simulink library "csc_tup_time_update_lib"  (R2014b)
settings: Solver=ode45  SolverMode=SingleTasking  StartTime=0.0  StopTime=10.0  RelTol=1e-3
undefined symbols (not defined in the file or in its folder): fcv_initializing
libraries: simulink x1, util_info_lib x1, csc_fcv_filter_convergence_lib x1, csu_itu_inertial_time_update_lib x1, csu_ttu_topo_time_update_lib x1, util_common_lib x1
settings Model: ExtModeAutoUpdateStatusClock=off  Creator=escrane  LastModifiedBy=mstewart

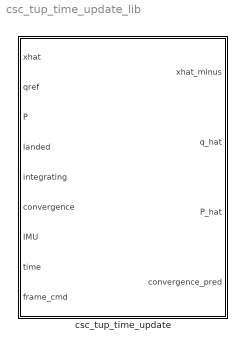
== system csc_tup_time_update_lib ==
  csc_tup_time_update : Subsystem

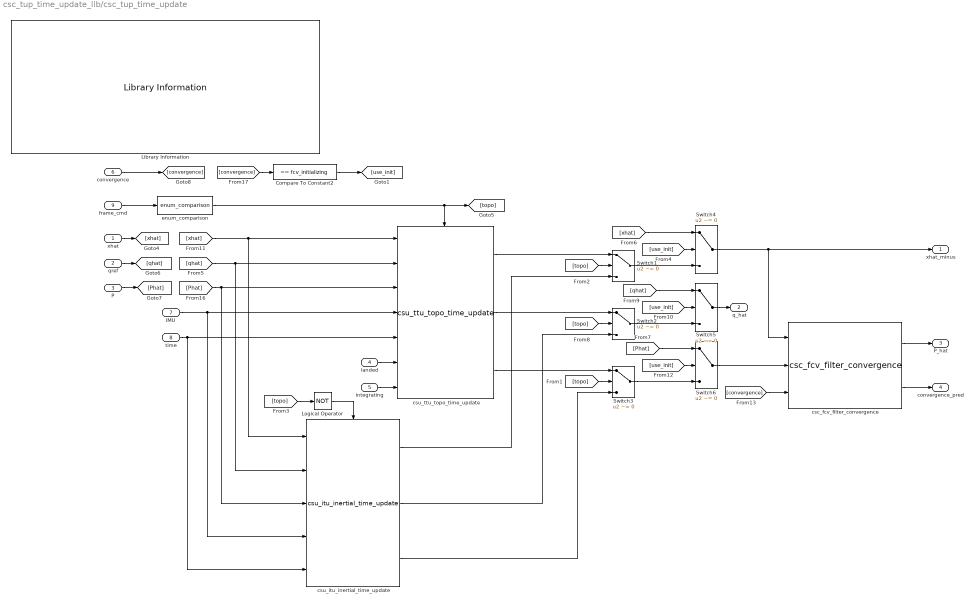
== system csc_tup_time_update_lib/csc_tup_time_update ==
  xhat : Inport
  qref : Inport  Port=2
  P : Inport  Port=3
  landed : Inport  Port=4
  integrating : Inport  Port=5
  convergence : Inport  Port=6
  IMU : Inport  Port=7
  time : Inport  Port=8
  frame_cmd : Inport  Port=9
  Compare To Constant2 : simulink/Logic and Bit Operations/Compare To Constant  relop===  const=fcv_initializing  OutDataTypeStr=boolean
  Library Information : util_info_lib/Library Information  owner='escrane'
  Logical Operator : Logic  Operator=NOT  AllPortsSameDT=off  OutDataTypeStr=boolean
  Switch{1..6} (6 alike) : Switch  Criteria=u2 ~= 0  Threshold=0.5  InputSameDT=on
  csc_fcv_filter_convergence : csc_fcv_filter_convergence_lib/csc_fcv_filter_convergence
  csu_itu_inertial_time_update : csu_itu_inertial_time_update_lib/csu_itu_inertial_time_update
  csu_ttu_topo_time_update : csu_ttu_topo_time_update_lib/csu_ttu_topo_time_update
  enum_comparison : util_common_lib/enum_comparison  comparison_type===
  xhat_minus : Outport
  q_hat : Outport  Port=2
  P_hat : Outport  Port=3
  convergence_pred : Outport  Port=4  OutDataTypeStr=double
  wires:
  integrating/1 -> csu_ttu_topo_time_update/7
  [convergence] -> csc_fcv_filter_convergence/3
  Switch6/1 -> csc_fcv_filter_convergence/2
  Switch5/1 -> q_hat/1
  [Phat] -> Switch6/1
  Switch3/1 -> Switch6/3
  [use_init] -> Switch6/2
  Switch2/1 -> Switch5/3
  [qhat] -> Switch5/1
  [use_init] -> Switch5/2
  [xhat] -> Switch4/1
  P/1 -> [Phat]
  qref/1 -> [qhat]
  xhat/1 -> [xhat]
  [use_init] -> Switch4/2
  Compare To Constant2/1 -> [use_init]
  Switch1/1 -> Switch4/3
  [convergence] -> Compare To Constant2/1
  convergence/1 -> [convergence]
  [topo] -> Switch3/2
  [topo] -> Switch2/2
  [topo] -> Switch1/2
  csc_fcv_filter_convergence/2 -> convergence_pred/1
  csc_fcv_filter_convergence/1 -> P_hat/1
  landed/1 -> csu_ttu_topo_time_update/6
  frame_cmd/1 -> enum_comparison/1
  enum_comparison/1 -> [topo], csu_ttu_topo_time_update/Enable
  Logical Operator/1 -> csu_itu_inertial_time_update/Enable
  time/1 -> csu_ttu_topo_time_update/5, csu_itu_inertial_time_update/5
  [xhat] -> csu_ttu_topo_time_update/1, csu_itu_inertial_time_update/1
  [qhat] -> csu_ttu_topo_time_update/2, csu_itu_inertial_time_update/2
  [Phat] -> csu_ttu_topo_time_update/3, csu_itu_inertial_time_update/3
  IMU/1 -> csu_ttu_topo_time_update/4, csu_itu_inertial_time_update/4
  csu_ttu_topo_time_update/1 -> Switch1/1
  csu_ttu_topo_time_update/2 -> Switch2/1
  csu_ttu_topo_time_update/3 -> Switch3/1
  Switch4/1 -> xhat_minus/1, csc_fcv_filter_convergence/1
  [topo] -> Logical Operator/1
  csu_itu_inertial_time_update/1 -> Switch1/3
  csu_itu_inertial_time_update/2 -> Switch2/3
  csu_itu_inertial_time_update/3 -> Switch3/3
